simulink model "MemoryBlock"  (R2024a)
settings: Solver=FixedStepDiscrete  StartTime=0.0  StopTime=10.0  FixedStep=0.1  RelTol=1e-3
settings Model: Creator=amir  LastModifiedBy=amir

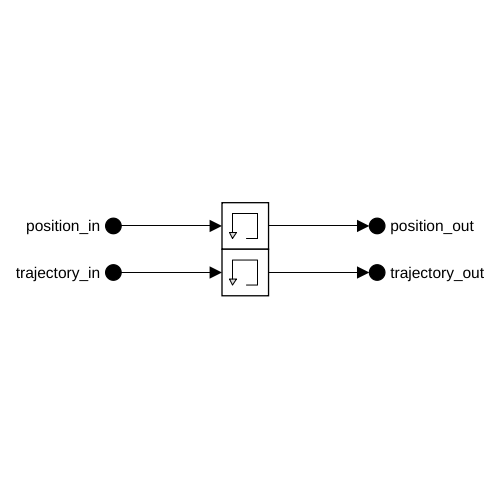
[thumbnail: Simulink's stored preview of the top-level diagram]
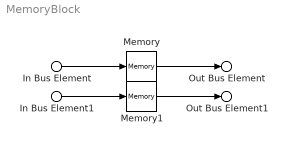
== system MemoryBlock ==
  In Bus Element : Inport  PortName=position_in
  In Bus Element1 : Inport  Port=2  PortName=trajectory_in
  Memory : Memory  LinearizeMemory=on  LinearizeAsDelay=on
  Memory1 : Memory  LinearizeMemory=on  LinearizeAsDelay=on
  Out Bus Element : Outport  PortName=position_out
  Out Bus Element1 : Outport  Port=2  PortName=trajectory_out
  wires:
  In Bus Element/1 -> Memory/1
  Memory/1 -> Out Bus Element/1
  In Bus Element1/1 -> Memory1/1
  Memory1/1 -> Out Bus Element1/1
